simulink model "FIRFilterDesign"  (R2020a)
settings: Solver=VariableStepAuto  StartTime=0.0  StopTime=10.0  RelTol=1e-3
settings Model: Creator=Hp  LastModifiedBy=Hp

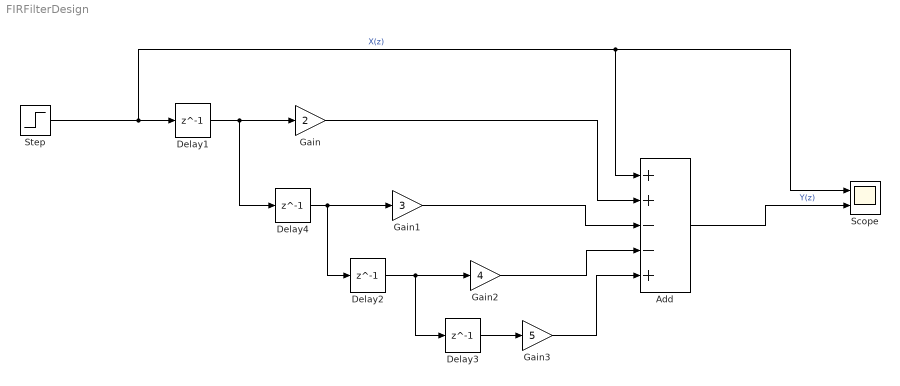
== system FIRFilterDesign ==
  Add : Sum  Inputs=++--+
  Delay{1..4} (4 alike) : Delay  DelayLength=1
  Gain : Gain  Gain=2
  Gain1 : Gain  Gain=3
  Gain2 : Gain  Gain=4
  Gain3 : Gain  Gain=5
  Scope : Scope  NumInputPorts=2
  Step : Step  SampleTime=0.1
  wires:
  Step/1 -> Scope/1, Add/1, Delay1/1  "X(z)"
  Delay1/1 -> Delay4/1, Gain/1
  Delay4/1 -> Delay2/1, Gain1/1
  Delay2/1 -> Delay3/1, Gain2/1
  Gain/1 -> Add/2
  Gain1/1 -> Add/3
  Gain2/1 -> Add/4
  Gain3/1 -> Add/5
  Add/1 -> Scope/2  "Y(z)"
  Delay3/1 -> Gain3/1
